simulink model "Greenhouse_3rdPoint_a"  (R2022a)
settings: Solver=VariableStepAuto  StartTime=0.0  StopTime=86400  RelTol=1e-3
undefined symbols (not defined in the file or in its folder): C_f1, C_f2, kaf1, kaf2, kaf_int, q_star_m1, q_star_m2, theta0_a, Ts, var_wf1, var_wf2
settings Model: Creator=loren  LastModifiedBy=leonardogiacobbe
settings ModelReferenceCC: EnableRefExpFcnMdlSchedulingChecks=off
settings RTWCC: Description=Generic Real-Time Target  GPUComputeCapability=5.0

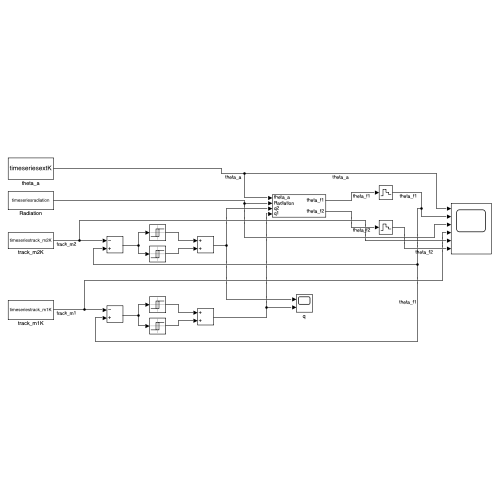
[thumbnail: Simulink's stored preview of the top-level diagram]
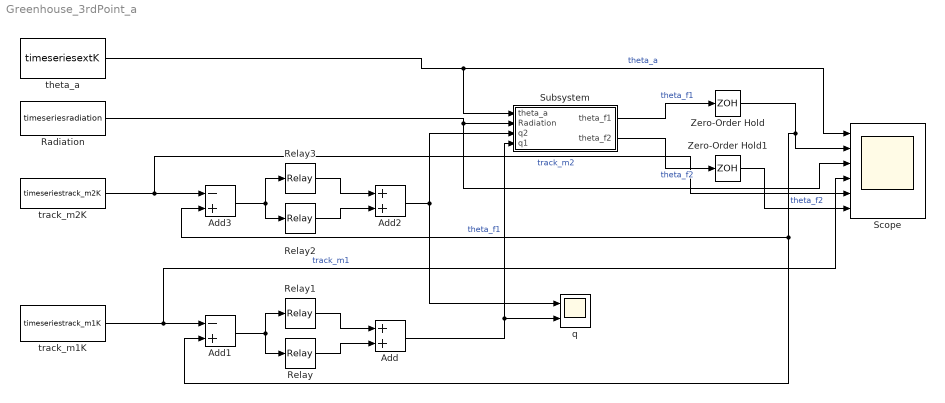
== system Greenhouse_3rdPoint_a ==
  Add : Sum
  Add1 : Sum  Inputs=-+
  Add2 : Sum
  Add3 : Sum  Inputs=-+
  Radiation : FromWorkspace  VariableName=timeseriesradiation  SampleTime=Ts
  Relay : Relay  OnSwitchValue=-1  OffSwitchValue=-1  OnOutputValue=-q_star_m1/2  OffOutputValue=q_star_m1/2
  Relay1 : Relay  OnSwitchValue=1  OffSwitchValue=1  OnOutputValue=-q_star_m1/2  OffOutputValue=q_star_m1/2
  Relay2 : Relay  OnSwitchValue=-1  OffSwitchValue=-1  OnOutputValue=-q_star_m2/2  OffOutputValue=q_star_m2/2
  Relay3 : Relay  OnSwitchValue=1  OffSwitchValue=1  OnOutputValue=-q_star_m2/2  OffOutputValue=q_star_m2/2
  Scope : Scope  NumInputPorts=6
  Subsystem : Subsystem
  Zero-Order Hold : ZeroOrderHold  SampleTime=Ts
  Zero-Order Hold1 : ZeroOrderHold  SampleTime=Ts
  q : Scope  NumInputPorts=2
  theta_a : FromWorkspace  VariableName=timeseriesextK  SampleTime=Ts
  track_m1K : FromWorkspace  VariableName=timeseriestrack_m1K  SampleTime=Ts
  track_m2K : FromWorkspace  VariableName=timeseriestrack_m2K  SampleTime=Ts
  wires:
  Subsystem/2(theta_f2) -> Zero-Order Hold1/1  "theta_f2"
  Radiation/1 -> Scope/3, Subsystem/2(Radiation)
  Zero-Order Hold1/1 -> Scope/6  "theta_f2"
  Subsystem/1(theta_f1) -> Zero-Order Hold/1  "theta_f1"
  Zero-Order Hold/1 -> Scope/2, Add3/2, Add1/2  "theta_f1"
  theta_a/1 -> Scope/1, Subsystem/1(theta_a)  "theta_a"
  Add2/1 -> Subsystem/3(q2), q/1
  Relay1/1 -> Add/1
  Relay/1 -> Add/2
  Add/1 -> q/2, Subsystem/4(q1)
  track_m1K/1 -> Scope/4, Add1/1  "track_m1"
  Add1/1 -> Relay/1, Relay1/1
  Relay3/1 -> Add2/1
  Relay2/1 -> Add2/2
  Add3/1 -> Relay3/1, Relay2/1
  track_m2K/1 -> Scope/5, Add3/1  "track_m2"

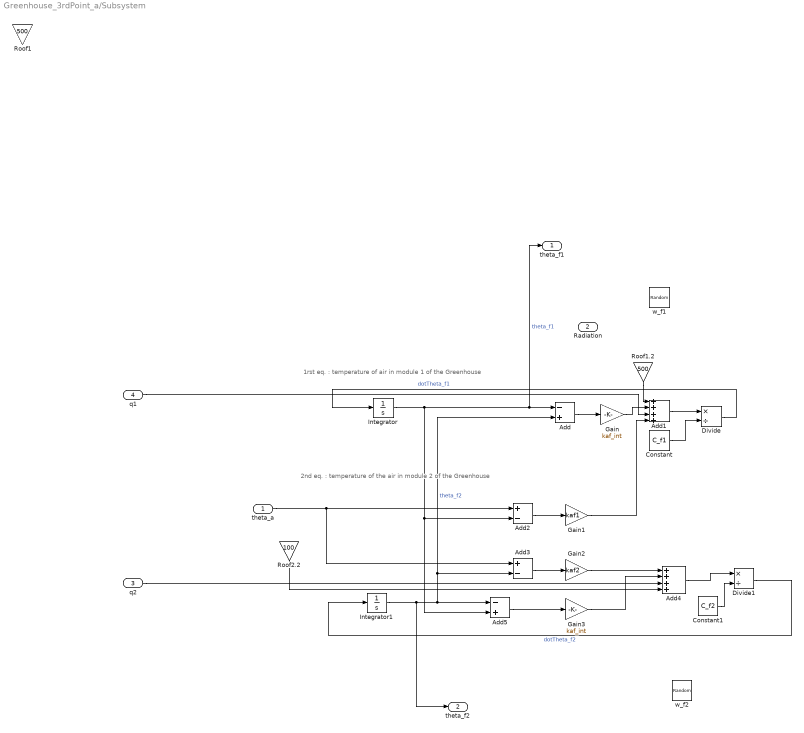
== system Greenhouse_3rdPoint_a/Subsystem ==
  note: 2nd eq. : temperature of the air in module 2 of the Greenhouse
  note: 1rst eq. : temperature of air in module 1 of the Greenhouse
  theta_a : Inport
  Radiation : Inport  Port=2
  q2 : Inport  Port=3
  q1 : Inport  Port=4
  Add : Sum  Inputs=-+
  Add1 : Sum  Inputs=++++
  Add2 : Sum  Inputs=+-
  Add3 : Sum  Inputs=+-
  Add4 : Sum  Inputs=++++
  Add5 : Sum  Inputs=-+
  Constant : Constant  Value=C_f1
  Constant1 : Constant  Value=C_f2
  Divide : Product  Inputs=*/
  Divide1 : Product  Inputs=*/
  Gain : Gain  Gain=kaf_int
  Gain1 : Gain  Gain=kaf1
  Gain2 : Gain  Gain=kaf2
  Gain3 : Gain  Gain=kaf_int
  Integrator : Integrator  InitialCondition=theta0_a
  Integrator1 : Integrator  InitialCondition=theta0_a
  Roof1 : Gain  Gain=500
  Roof1.2 : Gain  Gain=500
  Roof2.2 : Gain  Gain=100
  w_f1 : RandomNumber  Variance=var_wf1  SampleTime=Ts
  w_f2 : RandomNumber  Variance=var_wf2  SampleTime=Ts
  theta_f1 : Outport
  theta_f2 : Outport  Port=2
  wires:
  Add/1 -> Gain/1
  Gain1/1 -> Add1/4
  Add5/1 -> Gain3/1
  Add4/1 -> Divide1/1
  Integrator1/1 -> theta_f2/1, Add3/2, Add/2, Add5/1  "theta_f2"
  Divide1/1 -> Integrator1/1  "dotTheta_f2"
  Gain/1 -> Add1/2
  Constant/1 -> Divide/2
  Add1/1 -> Divide/1
  Add2/1 -> Gain1/1
  Add3/1 -> Gain2/1
  theta_a/1 -> Add3/1, Add2/1
  Integrator/1 -> Add5/2, Add2/2, theta_f1/1, Add/1  "theta_f1"
  Divide/1 -> Integrator/1  "dotTheta_f1"
  Gain3/1 -> Add4/2
  Gain2/1 -> Add4/1
  Constant1/1 -> Divide1/2
  Roof1.2/1 -> Add1/1
  Roof2.2/1 -> Add4/4
  q1/1 -> Add1/3
  q2/1 -> Add4/3
